simulink model "tftest_sl"  (R2024a)
settings: Solver=VariableStepAuto  StartTime=0.0  StopTime=10.0  RelTol=1e-3
values from neighbouring files (symbols this model uses):
  a = 1/tau    [mt_test.m]    (also in mtpractice_3.m = 4; tftest.m = 14)
  b = B    (= 18)    [tftest.m]
  c = C + 30    (= 48)    [tftest.m]
  d = D + 30    (= 46)    [tftest.m]
  f = F + 20    (= 37)    [tftest.m]
  g = G + 10    (= 28)    [tftest.m]
  h = H + 10    (= 25)    [tftest.m]
settings Model: Creator=yiche  LastModifiedBy=yiche

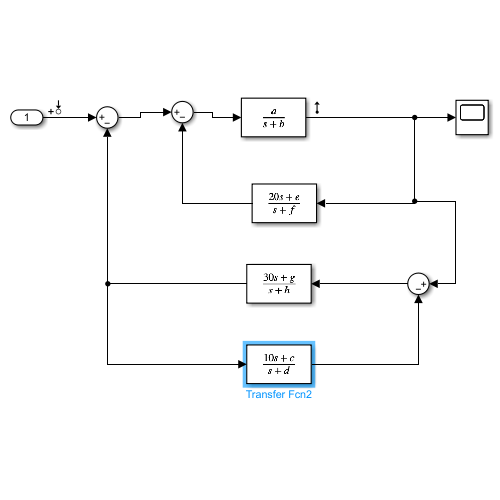
[thumbnail: Simulink's stored preview of the top-level diagram]
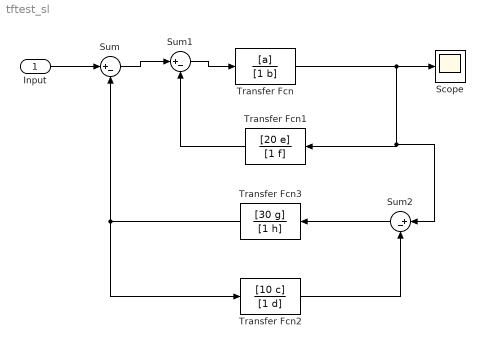
== system tftest_sl ==
  Input : Inport
  Scope : Scope
  Sum : Sum  Inputs=|+-
  Sum1 : Sum  Inputs=|+-
  Sum2 : Sum  Inputs=|+-
  Transfer Fcn : TransferFcn  Numerator=[a]  Denominator=[1 b]
  Transfer Fcn1 : TransferFcn  Numerator=[20 e]  Denominator=[1 f]
  Transfer Fcn2 : TransferFcn  Numerator=[10 c]  Denominator=[1 d]
  Transfer Fcn3 : TransferFcn  Numerator=[30 g]  Denominator=[1 h]
  wires:
  Input/1 -> Sum/1
  Sum/1 -> Sum1/1
  Sum1/1 -> Transfer Fcn/1
  Transfer Fcn1/1 -> Sum1/2
  Transfer Fcn3/1 -> Transfer Fcn2/1, Sum/2
  Sum2/1 -> Transfer Fcn3/1
  Transfer Fcn2/1 -> Sum2/2
  Transfer Fcn/1 -> Sum2/1, Transfer Fcn1/1, Scope/1
